simulink model "Four_DG_MG_PrimaryOnly"  (R2021b)
settings: Solver=ode23tb  StartTime=0.0  StopTime=5  RelTol=1e-3
model workspace (MAT data in the model file):
  Ts : Simulink.Parameter (value not decoded)
  secondary_on : Simulink.Parameter (value not decoded)
values from neighbouring files (symbols this model uses):
  a12 = 0    [Four_DG_MG_PrimaryOnlyScript.m]    (also in MPC_MG_script_raw_dmpc.m; MPC_MG_secondary_script.m)
  a14 = 0    [Four_DG_MG_PrimaryOnlyScript.m]    (also in MPC_MG_script_raw_dmpc.m; MPC_MG_secondary_script.m)
  a21 = 1    [Four_DG_MG_PrimaryOnlyScript.m]    (also in MPC_MG_script_raw_dmpc.m; MPC_MG_secondary_script.m)
  a23 = 0    [Four_DG_MG_PrimaryOnlyScript.m]    (also in MPC_MG_script_raw_dmpc.m; MPC_MG_secondary_script.m)
  a32 = 1    [Four_DG_MG_PrimaryOnlyScript.m]    (also in MPC_MG_script_raw_dmpc.m; MPC_MG_secondary_script.m)
  a34 = 0    [Four_DG_MG_PrimaryOnlyScript.m]    (also in MPC_MG_script_raw_dmpc.m; MPC_MG_secondary_script.m)
  a41 = 1    [Four_DG_MG_PrimaryOnlyScript.m]    (also in MPC_MG_script_raw_dmpc.m; MPC_MG_secondary_script.m)
  a43 = 0    [Four_DG_MG_PrimaryOnlyScript.m]    (also in MPC_MG_script_raw_dmpc.m; MPC_MG_secondary_script.m)
  b1v = 1    [Four_DG_MG_PrimaryOnlyScript.m]    (also in MPC_MG_script_raw_dmpc.m; MPC_MG_secondary_script.m; MPG_MG_July.m; MPG_MG_freq_script.m)
  b1w = 1    [Four_DG_MG_PrimaryOnlyScript.m]    (also in MPC_MG_script_raw_dmpc.m; MPC_MG_secondary_script.m; MPG_MG_July.m; MPG_MG_freq_script.m)
  b2v = 0    [Four_DG_MG_PrimaryOnlyScript.m]    (also in MPC_MG_script_raw_dmpc.m; MPC_MG_secondary_script.m; MPG_MG_July.m; MPG_MG_freq_script.m)
  b2w = 0    [Four_DG_MG_PrimaryOnlyScript.m]    (also in MPC_MG_script_raw_dmpc.m; MPC_MG_secondary_script.m; MPG_MG_July.m; MPG_MG_freq_script.m)
  b3v = 0    [Four_DG_MG_PrimaryOnlyScript.m]    (also in MPC_MG_script_raw_dmpc.m; MPC_MG_secondary_script.m; MPG_MG_July.m; MPG_MG_freq_script.m)
  b3w = 0    [Four_DG_MG_PrimaryOnlyScript.m]    (also in MPC_MG_script_raw_dmpc.m; MPC_MG_secondary_script.m; MPG_MG_July.m; MPG_MG_freq_script.m)
  b4v = 0    [Four_DG_MG_PrimaryOnlyScript.m]    (also in MPC_MG_script_raw_dmpc.m; MPC_MG_secondary_script.m; MPG_MG_July.m; MPG_MG_freq_script.m)
  b4w = 0    [Four_DG_MG_PrimaryOnlyScript.m]    (also in MPC_MG_script_raw_dmpc.m; MPC_MG_secondary_script.m; MPG_MG_July.m; MPG_MG_freq_script.m)
  C_f = 50e-6    (= 5e-05)    [Four_DG_MG_PrimaryOnlyScript.m]    (also in MPC_MG_script.m; MPC_MG_script_raw_dmpc.m; MPC_MG_secondary_script.m; MPG_MG_July.m)
  cf = 60    [Four_DG_MG_PrimaryOnlyScript.m]    (also in MPC_MG_script_raw_dmpc.m = 40; MPC_MG_secondary_script.m = 40; MPG_MG_July.m = 100; MPG_MG_freq_script.m = 100)
  cv = 60    [Four_DG_MG_PrimaryOnlyScript.m]    (also in MPC_MG_script_raw_dmpc.m = 40; MPC_MG_secondary_script.m = 40; MPG_MG_July.m = 100; MPG_MG_freq_script.m = 100)
  F = 1    [Four_DG_MG_PrimaryOnlyScript.m]    (also in dmpc.m = zeros(9,1))
  K_i1 = 420    [Four_DG_MG_PrimaryOnlyScript.m]
  K_i2 = K_i1    (= 420)    [Four_DG_MG_PrimaryOnlyScript.m]
  K_i3 = 390    [Four_DG_MG_PrimaryOnlyScript.m]
  K_i4 = K_i3    (= 390)    [Four_DG_MG_PrimaryOnlyScript.m]
  K_ii1 = 5e3    (= 5000)    [Four_DG_MG_PrimaryOnlyScript.m]
  K_ii2 = K_ii1    (= 5000)    [Four_DG_MG_PrimaryOnlyScript.m]
  K_ii3 = 16e3    (= 16000)    [Four_DG_MG_PrimaryOnlyScript.m]
  K_ii4 = K_ii3    (= 16000)    [Four_DG_MG_PrimaryOnlyScript.m]
  K_p1 = 0.1    [Four_DG_MG_PrimaryOnlyScript.m]
  K_p2 = K_p1    (= 0.1)    [Four_DG_MG_PrimaryOnlyScript.m]
  K_p3 = 0.05    [Four_DG_MG_PrimaryOnlyScript.m]
  K_p4 = K_p3    (= 0.05)    [Four_DG_MG_PrimaryOnlyScript.m]
  K_pi1 = 5    [Four_DG_MG_PrimaryOnlyScript.m]
  K_pi2 = K_pi1    (= 5)    [Four_DG_MG_PrimaryOnlyScript.m]
  K_pi3 = 10.5    [Four_DG_MG_PrimaryOnlyScript.m]
  K_pi4 = K_pi3    (= 10.5)    [Four_DG_MG_PrimaryOnlyScript.m]
  L_f = 1.35e-3    (= 0.00135)    [Four_DG_MG_PrimaryOnlyScript.m]    (also in MPC_MG_script.m; MPC_MG_script_raw_dmpc.m; MPC_MG_secondary_script.m; MPG_MG_July.m)
  L_in1 = 0.35e-3    (= 0.00035)    [Four_DG_MG_PrimaryOnlyScript.m]    (also in MPC_MG_script.m; MPC_MG_script_raw_dmpc.m; MPC_MG_secondary_script.m; MPG_MG_July.m)
  L_in2 = 0.35e-3    (= 0.00035)    [Four_DG_MG_PrimaryOnlyScript.m]    (also in MPC_MG_script.m; MPC_MG_script_raw_dmpc.m; MPC_MG_secondary_script.m; MPG_MG_July.m)
  L_in3 = 0.35e-3    (= 0.00035)    [Four_DG_MG_PrimaryOnlyScript.m]    (also in MPC_MG_script.m; MPC_MG_script_raw_dmpc.m; MPC_MG_secondary_script.m; MPG_MG_July.m)
  L_in4 = 0.35e-3    (= 0.00035)    [Four_DG_MG_PrimaryOnlyScript.m]    (also in MPC_MG_script.m; MPC_MG_script_raw_dmpc.m; MPC_MG_secondary_script.m; MPG_MG_July.m)
  lo_co = 0.2    [Four_DG_MG_PrimaryOnlyScript.m]    (also in MPC_MG_script.m = 0.05; MPC_MG_script_raw_dmpc.m; MPC_MG_secondary_script.m = 0.08; MPG_MG_July.m = 0.15)
  m_p1 = 9.4e-5/droopDivide    (= 9.4e-05)    [Four_DG_MG_PrimaryOnlyScript.m]    (also in MPC_MG_script.m; MPC_MG_script_raw_dmpc.m; MPC_MG_secondary_script.m; MPG_MG_July.m)
  m_p2 = 9.4e-5/droopDivide    (= 9.4e-05)    [Four_DG_MG_PrimaryOnlyScript.m]    (also in MPC_MG_script.m; MPC_MG_script_raw_dmpc.m; MPC_MG_secondary_script.m; MPG_MG_July.m)
  m_p3 = 12.5e-5/droopDivide    (= 0.000125)    [Four_DG_MG_PrimaryOnlyScript.m]    (also in MPC_MG_script.m; MPC_MG_script_raw_dmpc.m; MPC_MG_secondary_script.m; MPG_MG_July.m)
  m_p4 = 12.5e-5/droopDivide    (= 0.000125)    [Four_DG_MG_PrimaryOnlyScript.m]    (also in MPC_MG_script.m; MPC_MG_script_raw_dmpc.m; MPC_MG_secondary_script.m; MPG_MG_July.m)
  n_q1 = 1.3e-3/droopDivide2    (= 0.00013)    [Four_DG_MG_PrimaryOnlyScript.m]    (also in MPC_MG_script.m; MPC_MG_script_raw_dmpc.m; MPC_MG_secondary_script.m; MPG_MG_July.m)
  n_q2 = 1.3e-3/droopDivide2    (= 0.00013)    [Four_DG_MG_PrimaryOnlyScript.m]    (also in MPC_MG_script.m; MPC_MG_script_raw_dmpc.m; MPC_MG_secondary_script.m; MPG_MG_July.m)
  n_q3 = 1.5e-3/droopDivide2    (= 0.00015)    [Four_DG_MG_PrimaryOnlyScript.m]    (also in MPC_MG_script.m; MPC_MG_script_raw_dmpc.m; MPC_MG_secondary_script.m; MPG_MG_July.m)
  n_q4 = 1.5e-3/droopDivide2    (= 0.00015)    [Four_DG_MG_PrimaryOnlyScript.m]    (also in MPC_MG_script.m; MPC_MG_script_raw_dmpc.m; MPC_MG_secondary_script.m; MPG_MG_July.m)
  pq_gain = 3/2    (= 1.5)    [Four_DG_MG_PrimaryOnlyScript.m]
  R_f = 0.1    [Four_DG_MG_PrimaryOnlyScript.m]    (also in MPC_MG_script.m; MPC_MG_script_raw_dmpc.m; MPC_MG_secondary_script.m; MPG_MG_July.m)
  R_in1 = 0.03    [Four_DG_MG_PrimaryOnlyScript.m]    (also in MPC_MG_script.m; MPC_MG_script_raw_dmpc.m; MPC_MG_secondary_script.m; MPG_MG_July.m)
  R_in2 = 0.03    [Four_DG_MG_PrimaryOnlyScript.m]    (also in MPC_MG_script.m; MPC_MG_script_raw_dmpc.m; MPC_MG_secondary_script.m; MPG_MG_July.m)
  R_in3 = 0.03    [Four_DG_MG_PrimaryOnlyScript.m]    (also in MPC_MG_script.m; MPC_MG_script_raw_dmpc.m; MPC_MG_secondary_script.m; MPG_MG_July.m)
  R_in4 = 0.03    [Four_DG_MG_PrimaryOnlyScript.m]    (also in MPC_MG_script.m; MPC_MG_script_raw_dmpc.m; MPC_MG_secondary_script.m; MPG_MG_July.m)
  secondary = 1    [Four_DG_MG_PrimaryOnlyScript.m]
  secondary2 = 1    [Four_DG_MG_PrimaryOnlyScript.m]
  time_thresh = 0.6    [Four_DG_MG_PrimaryOnlyScript.m]    (also in MPC_MG_script_raw_dmpc.m = 1.5; MPC_MG_secondary_script.m = 2; MPG_MG_July.m = 0.5; MPG_MG_freq_script.m = 0.5)
  Ts = 10e-6    (= 1e-05)    [Four_DG_MG_PrimaryOnlyScript.m]    (also in MPC_MG_script.m; MPC_MG_script_raw_dmpc.m; MPC_MG_secondary_script.m; MPG_MG_July.m)
  V_nom = 220*sqrt(2)    [Four_DG_MG_PrimaryOnlyScript.m]    (also in MPC_MG_script.m; MPC_MG_script_raw_dmpc.m; MPC_MG_secondary_script.m; MPG_MG_July.m)
  Vdc = 600    [Four_DG_MG_PrimaryOnlyScript.m]    (also in MPC_MG_script.m; MPC_MG_script_raw_dmpc.m; MPC_MG_secondary_script.m; MPG_MG_July.m)
  w_nom = 2*pi*50    (= 314.159265359)    [Four_DG_MG_PrimaryOnlyScript.m]    (also in MPC_MG_script.m; MPC_MG_script_raw_dmpc.m; MPC_MG_secondary_script.m; MPG_MG_July.m)
undefined symbols (not defined in the file or in its folder): K_d
libraries: slpidlib x16, spsThreePhaseSeriesRLCBranchLib x15, spsabctodq0Lib x13, spsThreePhaseVIMeasurementLib x12, eeGeneralControl x8, spsOnDelayLib x8, spsPMUPLLBasedPositiveSequenceLib x4, eePwmGeneratorTwoLevel x4, spsdq0toabcLib x4, spsDCVoltageSourceLib x4, spsSeriesRLCBranchLib x4, spsTwoLevelConverterLib x4
(part 2 of 4)

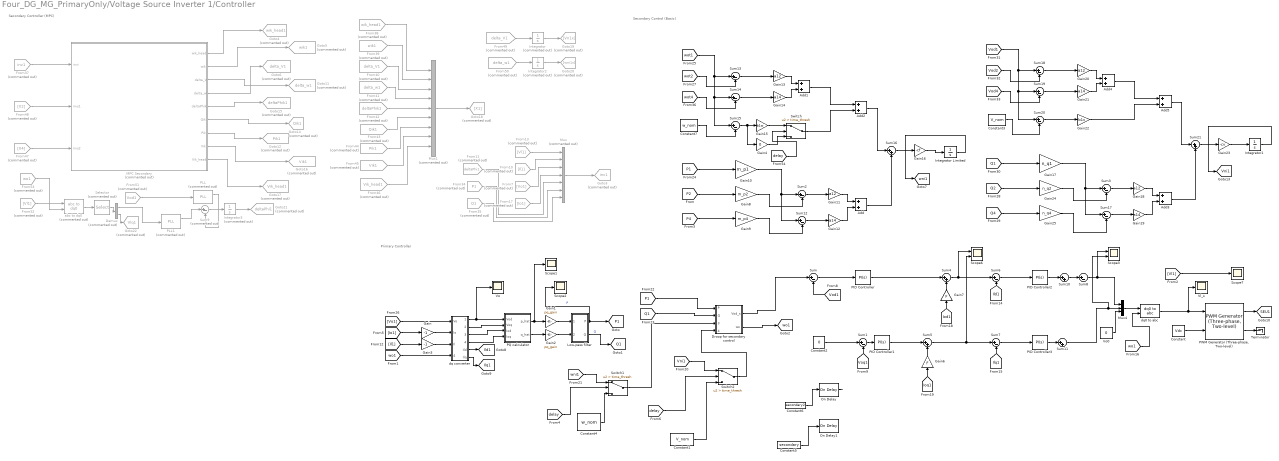
== system Four_DG_MG_PrimaryOnly/Voltage Source Inverter 1/Controller ==
  note: Secondary Controller (MPC)
  note: Secondary Control (Basic)
  note: Primary Controller
  Add{,1..5} (6 alike) : Sum
  Constant : Constant  Value=Vdc
  Constant1 : Constant  Value=V_nom
  Constant2 : Constant  Value=0
  Constant3 : Constant  Value=V_nom
  Constant4 : Constant  Value=w_nom
  Constant5 : Constant  Value=secondary
  Constant6 : Constant  Value=secondary2
  Constant7 : Constant  Value=w_nom
  Demux : Demux  Commented=on  Outputs=2
  Droop for secondary control : Subsystem
  From10 : From  Commented=on  GotoTag=Il1  TagVisibility=global
  From11 : From  Commented=on  GotoTag=deltaPhi1  TagVisibility=global
  From13 : From  Commented=on  GotoTag=Vl1  TagVisibility=global
  From17 : From  Commented=on  GotoTag=Io1  TagVisibility=global
  From34 : From  Commented=on  GotoTag=P1  TagVisibility=global
  From35 : From  Commented=on  GotoTag=Q1  TagVisibility=global
  From37 : From  Commented=on  GotoTag=inv1  TagVisibility=global
  From38 : From  Commented=on  GotoTag=wik_head1  TagVisibility=global
  From39 : From  Commented=on  GotoTag=wik1  TagVisibility=global
  From40 : From  Commented=on  GotoTag=delta_V1  TagVisibility=global
  From41 : From  Commented=on  GotoTag=delta_w1  TagVisibility=global
  From42 : From  Commented=on  GotoTag=deltaPhik1  TagVisibility=global
  From43 : From  Commented=on  GotoTag=Qik1  TagVisibility=global
  From44 : From  Commented=on  GotoTag=Pik1  TagVisibility=global
  From45 : From  Commented=on  GotoTag=Vik1  TagVisibility=global
  From46 : From  Commented=on  GotoTag=Vik_head1  TagVisibility=global
  From47 : From  Commented=on  GotoTag=X4
  From48 : From  Commented=on  GotoTag=X2
  From49 : From  Commented=on  GotoTag=delta_V1  TagVisibility=global
  From50 : From  Commented=on  GotoTag=delta_w1  TagVisibility=global
  From51 : From  Commented=on  GotoTag=Vod1  TagVisibility=global
  From52 : From  Commented=on  GotoTag=Vl1  TagVisibility=global
  From53 : From  Commented=on  GotoTag=wo1  TagVisibility=global
  From7 : From  Commented=on  GotoTag=Vo1  TagVisibility=global
  Gain : Gain  Gain=-1
  Gain1 : Gain  Gain=pq_gain
  Gain10 : Gain  Gain=m_p1
  Gain{11,13,18,20} (4 alike) : Gain  Gain=a12
  Gain{12,14,19,21} (4 alike) : Gain  Gain=a14
  Gain15 : Gain  Gain=b1w
  Gain16 : Gain  Gain=-cf
  Gain17 : Gain  Gain=n_q1
  Gain2 : Gain  Gain=pq_gain
  Gain22 : Gain  Gain=b1v
  Gain23 : Gain  Gain=-cv
  Gain24 : Gain  Gain=n_q2
  Gain25 : Gain  Gain=n_q4
  Gain3 : Gain  Gain=-1
  Gain4 : Gain  Gain=0
  Gain6 : Gain  Gain=F
  Gain7 : Gain  Gain=F
  Gain8 : Gain  Gain=m_p2
  Gain9 : Gain  Gain=m_p4
  Goto11 : Goto  Commented=on  GotoTag=delta_w1  TagVisibility=global
  Goto12 : Goto  Commented=on  GotoTag=Pik1  TagVisibility=global
  Goto14 : Goto  Commented=on  GotoTag=Qik1  TagVisibility=global
  Goto15 : Goto  Commented=on  GotoTag=deltaPhik1  TagVisibility=global
  Goto16 : Goto  Commented=on  GotoTag=Vik1  TagVisibility=global
  Goto17 : Goto  Commented=on  GotoTag=Vik_head1  TagVisibility=global
  Goto18 : Goto  Commented=on  GotoTag=X1
  Goto19 : Goto  Commented=on  GotoTag=Vn1x
  Goto20 : Goto  Commented=on  GotoTag=wni1x
  Goto21 : Goto  Commented=on  GotoTag=deltaPhi1  TagVisibility=global
  Goto22 : Goto  Commented=on  GotoTag=Vlq1  TagVisibility=global
  Goto3 : Goto  Commented=on  GotoTag=inv1  TagVisibility=global
  Goto4 : Goto  Commented=on  GotoTag=wik_head1  TagVisibility=global
  Goto5 : Goto  Commented=on  GotoTag=wik1  TagVisibility=global
  Goto6 : Goto  Commented=on  GotoTag=delta_V1  TagVisibility=global
  Integrator : Integrator  Commented=on
  Integrator Limited : Integrator  InitialCondition=50*2*pi  UpperSaturationLimit=51*2*pi  LowerSaturationLimit=50*2*pi
  Integrator1 : Integrator  InitialCondition=311  UpperSaturationLimit=373.35  LowerSaturationLimit=248.90
  Integrator2 : Integrator  Commented=on
  Integrator3 : Integrator  Commented=on
  Low-pass filter : Subsystem
  "MPC Secondary  " : MATLAB Function  Commented=on  TreatAsAtomicUnit=on
  Mux : Mux  Commented=on  Inputs=7
  Mux1 : Mux  Commented=on  Inputs=9
  Mux4 : Mux  Inputs=3
  On Delay : spsOnDelayLib/On Delay  DelayType=On delay  delay=4  ic=0  Ts=0
      settings: SourceProductBaseCode=PS
  On Delay1 : spsOnDelayLib/On Delay  DelayType=On delay  delay=4  ic=0  Ts=0
      settings: SourceProductBaseCode=PS
  PID Controller : slpidlib/PID Controller  Controller=PI  Form=Parallel  TimeDomain=Continuous-time  UseExternalTs=off  SampleTime=-1  IntegratorMethod=Forward Euler  FilterMethod=Forward Euler  ControllerParametersSource=internal  P=K_p1  I=K_i1  D=K_d  UseFilter=on  N=100  TunerSelectOption=Frequency Response Based  InitialConditionSource=internal  InitialConditionForIntegrator=0  InitialConditionForFilter=0  DifferentiatorICPrevScaledInput=0  ExternalReset=none  TrackingMode=off  Kt=1  LimitOutput=off  SatLimitsSource=internal  UpperSaturationLimit=50  LowerSaturationLimit=-50  LinearizeAsGain=on  AntiWindupMode=none  Kb=1  POutMin=[]  POutMax=[]  IOutMin=[]  IOutMax=[]  DOutMin=[]  DOutMax=[]  NOutMin=[]  NOutMax=[]  SumOutMin=[]  SumOutMax=[]  SaturationOutMin=[]  SaturationOutMax=[]  PParamMin=[]  PParamMax=[]  IParamMin=[]  IParamMax=[]  DParamMin=[]  DParamMax=[]  NParamMin=[]  NParamMax=[]  KbParamMin=[]  KbParamMax=[]  KtParamMin=[]  KtParamMax=[]  KbOutMin=[]  KbOutMax=[]  KtOutMin=[]  KtOutMax=[]  IntegratorOutMin=[]  IntegratorOutMax=[]  FilterOutMin=[]  FilterOutMax=[]  SumI1OutMin=[]  SumI1OutMax=[]  SumI2OutMin=[]  SumI2OutMax=[]  SumI3OutMin=[]  SumI3OutMax=[]  SumI4OutMin=[]  SumI4OutMax=[]  SumDOutMin=[]  SumDOutMax=[]  DifferentiatorOutMin=[]  DifferentiatorOutMax=[]  FilterDiffOutCoefMin=[]  FilterDiffOutCoefMax=[]  ReciprocalOutMin=[]  ReciprocalOutMax=[]  SumDenOutMin=[]  SumDenOutMax=[]  SumNumOutMin=[]  SumNumOutMax=[]  DivideOutMin=[]  DivideOutMax=[]  UdiffTsProdOutMin=[]  UdiffTsProdOutMax=[]  NTsProdOutMin=[]  NTsProdOutMax=[]  UintegralTsProdOutMin=[]  UintegralTsProdOutMax=[]  UngainTsProdOutMin=[]  UngainTsProdOutMax=[]  IntegratorContinuousStateAttributes=''  IntegratorStateMustResolveToSignalObject=off  IntegratorRTWStateStorageClass=Auto  FilterContinuousStateAttributes=''  FilterStateMustResolveToSignalObject=off  FilterRTWStateStorageClass=Auto  ParallelPVariant=InternalParameters  IdealPVariant=Disabled  IVariant=InternalParameters  DVariant=Disabled  IntegratorVariant=Continuous  SatVariant=Disabled  AWVariant=Passthrough  PCopyVariant=Disabled  TRVariant=Disabled  FdbkBlocksVariant=Forward  IdealPFdbkVariant=Disabled  SatFdbkVariant=Disabled  DerivativeFilterVariant=Disabled  NVariant=Disabled  NCopyVariant=Disabled_SignalSpec  FilterICVariant=Disabled  IntegratorICVariant=InternalICs  ExternalResetVariant=Disabled  TRSumVariant=Passthrough  SumFdbkVariant=Disabled  SumVariant=Sum_PI  TsampFilterVariant=InternalTs  TsampNgainVariant=Passthrough  TsampIntegralVariant=Passthrough  ExternalSaturationOutDataTypeStr=Inherit: Same as second input
  PID Controller1 : slpidlib/PID Controller  Controller=PI  Form=Parallel  TimeDomain=Continuous-time  UseExternalTs=off  SampleTime=-1  IntegratorMethod=Forward Euler  FilterMethod=Forward Euler  ControllerParametersSource=internal  P=K_p1  I=K_i1  D=K_d  UseFilter=on  N=100  TunerSelectOption=Frequency Response Based  InitialConditionSource=internal  InitialConditionForIntegrator=0  InitialConditionForFilter=0  DifferentiatorICPrevScaledInput=0  ExternalReset=none  TrackingMode=off  Kt=1  LimitOutput=off  SatLimitsSource=internal  UpperSaturationLimit=50  LowerSaturationLimit=-50  LinearizeAsGain=on  AntiWindupMode=none  Kb=1  POutMin=[]  POutMax=[]  IOutMin=[]  IOutMax=[]  DOutMin=[]  DOutMax=[]  NOutMin=[]  NOutMax=[]  SumOutMin=[]  SumOutMax=[]  SaturationOutMin=[]  SaturationOutMax=[]  PParamMin=[]  PParamMax=[]  IParamMin=[]  IParamMax=[]  DParamMin=[]  DParamMax=[]  NParamMin=[]  NParamMax=[]  KbParamMin=[]  KbParamMax=[]  KtParamMin=[]  KtParamMax=[]  KbOutMin=[]  KbOutMax=[]  KtOutMin=[]  KtOutMax=[]  IntegratorOutMin=[]  IntegratorOutMax=[]  FilterOutMin=[]  FilterOutMax=[]  SumI1OutMin=[]  SumI1OutMax=[]  SumI2OutMin=[]  SumI2OutMax=[]  SumI3OutMin=[]  SumI3OutMax=[]  SumI4OutMin=[]  SumI4OutMax=[]  SumDOutMin=[]  SumDOutMax=[]  DifferentiatorOutMin=[]  DifferentiatorOutMax=[]  FilterDiffOutCoefMin=[]  FilterDiffOutCoefMax=[]  ReciprocalOutMin=[]  ReciprocalOutMax=[]  SumDenOutMin=[]  SumDenOutMax=[]  SumNumOutMin=[]  SumNumOutMax=[]  DivideOutMin=[]  DivideOutMax=[]  UdiffTsProdOutMin=[]  UdiffTsProdOutMax=[]  NTsProdOutMin=[]  NTsProdOutMax=[]  UintegralTsProdOutMin=[]  UintegralTsProdOutMax=[]  UngainTsProdOutMin=[]  UngainTsProdOutMax=[]  IntegratorContinuousStateAttributes=''  IntegratorStateMustResolveToSignalObject=off  IntegratorRTWStateStorageClass=Auto  FilterContinuousStateAttributes=''  FilterStateMustResolveToSignalObject=off  FilterRTWStateStorageClass=Auto  ParallelPVariant=InternalParameters  IdealPVariant=Disabled  IVariant=InternalParameters  DVariant=Disabled  IntegratorVariant=Continuous  SatVariant=Disabled  AWVariant=Passthrough  PCopyVariant=Disabled  TRVariant=Disabled  FdbkBlocksVariant=Forward  IdealPFdbkVariant=Disabled  SatFdbkVariant=Disabled  DerivativeFilterVariant=Disabled  NVariant=Disabled  NCopyVariant=Disabled_SignalSpec  FilterICVariant=Disabled  IntegratorICVariant=InternalICs  ExternalResetVariant=Disabled  TRSumVariant=Passthrough  SumFdbkVariant=Disabled  SumVariant=Sum_PI  TsampFilterVariant=InternalTs  TsampNgainVariant=Passthrough  TsampIntegralVariant=Passthrough  ExternalSaturationOutDataTypeStr=Inherit: Same as second input
  PID Controller2 : slpidlib/PID Controller  Controller=PI  Form=Parallel  TimeDomain=Continuous-time  UseExternalTs=off  SampleTime=-1  IntegratorMethod=Forward Euler  FilterMethod=Forward Euler  ControllerParametersSource=internal  P=K_pi1  I=K_ii1  D=K_d  UseFilter=on  N=100  TunerSelectOption=Frequency Response Based  InitialConditionSource=internal  InitialConditionForIntegrator=0  InitialConditionForFilter=0  DifferentiatorICPrevScaledInput=0  ExternalReset=none  TrackingMode=off  Kt=1  LimitOutput=off  SatLimitsSource=internal  UpperSaturationLimit=inf  LowerSaturationLimit=-inf  LinearizeAsGain=on  AntiWindupMode=none  Kb=1  POutMin=[]  POutMax=[]  IOutMin=[]  IOutMax=[]  DOutMin=[]  DOutMax=[]  NOutMin=[]  NOutMax=[]  SumOutMin=[]  SumOutMax=[]  SaturationOutMin=[]  SaturationOutMax=[]  PParamMin=[]  PParamMax=[]  IParamMin=[]  IParamMax=[]  DParamMin=[]  DParamMax=[]  NParamMin=[]  NParamMax=[]  KbParamMin=[]  KbParamMax=[]  KtParamMin=[]  KtParamMax=[]  KbOutMin=[]  KbOutMax=[]  KtOutMin=[]  KtOutMax=[]  IntegratorOutMin=[]  IntegratorOutMax=[]  FilterOutMin=[]  FilterOutMax=[]  SumI1OutMin=[]  SumI1OutMax=[]  SumI2OutMin=[]  SumI2OutMax=[]  SumI3OutMin=[]  SumI3OutMax=[]  SumI4OutMin=[]  SumI4OutMax=[]  SumDOutMin=[]  SumDOutMax=[]  DifferentiatorOutMin=[]  DifferentiatorOutMax=[]  FilterDiffOutCoefMin=[]  FilterDiffOutCoefMax=[]  ReciprocalOutMin=[]  ReciprocalOutMax=[]  SumDenOutMin=[]  SumDenOutMax=[]  SumNumOutMin=[]  SumNumOutMax=[]  DivideOutMin=[]  DivideOutMax=[]  UdiffTsProdOutMin=[]  UdiffTsProdOutMax=[]  NTsProdOutMin=[]  NTsProdOutMax=[]  UintegralTsProdOutMin=[]  UintegralTsProdOutMax=[]  UngainTsProdOutMin=[]  UngainTsProdOutMax=[]  IntegratorContinuousStateAttributes=''  IntegratorStateMustResolveToSignalObject=off  IntegratorRTWStateStorageClass=Auto  FilterContinuousStateAttributes=''  FilterStateMustResolveToSignalObject=off  FilterRTWStateStorageClass=Auto  ParallelPVariant=InternalParameters  IdealPVariant=Disabled  IVariant=InternalParameters  DVariant=Disabled  IntegratorVariant=Continuous  SatVariant=Disabled  AWVariant=Passthrough  PCopyVariant=Disabled  TRVariant=Disabled  FdbkBlocksVariant=Forward  IdealPFdbkVariant=Disabled  SatFdbkVariant=Disabled  DerivativeFilterVariant=Disabled  NVariant=Disabled  NCopyVariant=Disabled_SignalSpec  FilterICVariant=Disabled  IntegratorICVariant=InternalICs  ExternalResetVariant=Disabled  TRSumVariant=Passthrough  SumFdbkVariant=Disabled  SumVariant=Sum_PI  TsampFilterVariant=InternalTs  TsampNgainVariant=Passthrough  TsampIntegralVariant=Passthrough  ExternalSaturationOutDataTypeStr=Inherit: Same as second input
  PID Controller3 : slpidlib/PID Controller  Controller=PI  Form=Parallel  TimeDomain=Continuous-time  UseExternalTs=off  SampleTime=-1  IntegratorMethod=Forward Euler  FilterMethod=Forward Euler  ControllerParametersSource=internal  P=K_pi1  I=K_ii1  D=K_d  UseFilter=on  N=100  TunerSelectOption=Frequency Response Based  InitialConditionSource=internal  InitialConditionForIntegrator=0  InitialConditionForFilter=0  DifferentiatorICPrevScaledInput=0  ExternalReset=none  TrackingMode=off  Kt=1  LimitOutput=off  SatLimitsSource=internal  UpperSaturationLimit=inf  LowerSaturationLimit=-inf  LinearizeAsGain=on  AntiWindupMode=none  Kb=1  POutMin=[]  POutMax=[]  IOutMin=[]  IOutMax=[]  DOutMin=[]  DOutMax=[]  NOutMin=[]  NOutMax=[]  SumOutMin=[]  SumOutMax=[]  SaturationOutMin=[]  SaturationOutMax=[]  PParamMin=[]  PParamMax=[]  IParamMin=[]  IParamMax=[]  DParamMin=[]  DParamMax=[]  NParamMin=[]  NParamMax=[]  KbParamMin=[]  KbParamMax=[]  KtParamMin=[]  KtParamMax=[]  KbOutMin=[]  KbOutMax=[]  KtOutMin=[]  KtOutMax=[]  IntegratorOutMin=[]  IntegratorOutMax=[]  FilterOutMin=[]  FilterOutMax=[]  SumI1OutMin=[]  SumI1OutMax=[]  SumI2OutMin=[]  SumI2OutMax=[]  SumI3OutMin=[]  SumI3OutMax=[]  SumI4OutMin=[]  SumI4OutMax=[]  SumDOutMin=[]  SumDOutMax=[]  DifferentiatorOutMin=[]  DifferentiatorOutMax=[]  FilterDiffOutCoefMin=[]  FilterDiffOutCoefMax=[]  ReciprocalOutMin=[]  ReciprocalOutMax=[]  SumDenOutMin=[]  SumDenOutMax=[]  SumNumOutMin=[]  SumNumOutMax=[]  DivideOutMin=[]  DivideOutMax=[]  UdiffTsProdOutMin=[]  UdiffTsProdOutMax=[]  NTsProdOutMin=[]  NTsProdOutMax=[]  UintegralTsProdOutMin=[]  UintegralTsProdOutMax=[]  UngainTsProdOutMin=[]  UngainTsProdOutMax=[]  IntegratorContinuousStateAttributes=''  IntegratorStateMustResolveToSignalObject=off  IntegratorRTWStateStorageClass=Auto  FilterContinuousStateAttributes=''  FilterStateMustResolveToSignalObject=off  FilterRTWStateStorageClass=Auto  ParallelPVariant=InternalParameters  IdealPVariant=Disabled  IVariant=InternalParameters  DVariant=Disabled  IntegratorVariant=Continuous  SatVariant=Disabled  AWVariant=Passthrough  PCopyVariant=Disabled  TRVariant=Disabled  FdbkBlocksVariant=Forward  IdealPFdbkVariant=Disabled  SatFdbkVariant=Disabled  DerivativeFilterVariant=Disabled  NVariant=Disabled  NCopyVariant=Disabled_SignalSpec  FilterICVariant=Disabled  IntegratorICVariant=InternalICs  ExternalResetVariant=Disabled  TRSumVariant=Passthrough  SumFdbkVariant=Disabled  SumVariant=Sum_PI  TsampFilterVariant=InternalTs  TsampNgainVariant=Passthrough  TsampIntegralVariant=Passthrough  ExternalSaturationOutDataTypeStr=Inherit: Same as second input
  PLL : spsPLLLib/PLL  Commented=on  Fmin=45  Par_Init=[0, 60]  ParK=[180, 3200, 1]  TcD=1e-4  MaxRateChangeFreq=12  FilterCutOffFreq=25  Ts=0  AGC=on
      settings: SourceProductBaseCode=PS
  PLL1 : spsPLLLib/PLL  Commented=on  Fmin=45  Par_Init=[0, 60]  ParK=[180, 3200, 1]  TcD=1e-4  MaxRateChangeFreq=12  FilterCutOffFreq=25  Ts=0  AGC=on
      settings: SourceProductBaseCode=PS
  PQ calculator : Subsystem
  "PWM Generator (Three-phase, Two-level)" : eePwmGeneratorTwoLevel/PWM Generator (Three-phase, Two-level)  PWMMode=Continuous PWM (CPWM)  CPWMMode=SPWM: sinusoidal PWM  DPWMMode=60 DPWM: 60 degree discontinuous PWM  fsw=f_c  Ts=Ts
      settings: SourceProductBaseCode=PS
  Scope1 : Scope
  Scope2 : Scope
  Scope3 : Scope  NumInputPorts=2
  Scope6 : Scope  NumInputPorts=2
  Scope7 : Scope
  Selector : Selector  Commented=on  InputPortWidth=3  IndexOptions=Index vector (dialog)  Indices=[1 2]  OutputSizes=1
  Sum{,1..3,6..8,12..15,17..20} (15 alike) : Sum  Inputs=|+-
  Sum{4..5,10..11,16,21} (6 alike) : Sum  Inputs=|++
  Sum9 : Sum  Commented=on  Inputs=|+-
  Switch : Switch  Criteria=u2 > Threshold  Threshold=time_thresh
  Switch1 : Switch  Criteria=u2 > Threshold  Threshold=time_thresh
  Switch2 : Switch  Criteria=u2 > Threshold  Threshold=time_thresh
  Terminator : Terminator
  Vl_s : Scope
  Vo : Scope
  Vo0 : Constant  Value=0
  abc to dq0 : spsabctodq0Lib/abc to dq0  Commented=on  Alignment=90 degrees behind phase A axis
  dq converter : Subsystem
  dq0 to abc : spsdq0toabcLib/dq0 to abc  Alignment=90 degrees behind phase A axis
  tag scope: Ild1=global, Ilq1=global, P1=global, Q1=global, SEU1=global, Vni1=global, wni1=global, wo1=global
  wires:
  dq converter/1(Vod) -> Vo/1, PQ calculator/1(Vod)
  [Vl1] -> Scope7/1
  [Io1] -> Gain/1
  Sum/1 -> PID Controller/1
  dq converter/6(Ilq) -> [Ilq1]
  Sum1/1 -> PID Controller1/1
  Sum7/1 -> PID Controller3/1
  [Voq1] -> Sum1/2
  dq converter/5(Ild) -> [Ild1]
  Mux4/1 -> dq0 to abc/1
  PID Controller1/1 -> Sum5/1
  Vo0/1 -> Mux4/3
  Sum6/1 -> PID Controller2/1
  PID Controller/1 -> Sum4/1
  PQ calculator/1(p_hat) -> Gain1/1, Scope1/1
  [Il1] -> Gain3/1
  [Vo1] -> dq converter/1(Vo)
  Sum11/1 -> Scope3/2, Mux4/2
  Gain6/1 -> Sum5/2
  dq converter/4(Ioq) -> PQ calculator/4(Ioq)
  "PWM Generator (Three-phase, Two-level)"/2 -> Terminator/1
  Sum5/1 -> Sum7/1, Scope6/2
  Constant/1 -> "PWM Generator (Three-phase, Two-level)"/2
  dq converter/3(Iod) -> PQ calculator/3(Iod)
  dq converter/2(Voq) -> PQ calculator/2(Voq)
  Sum8/1 -> Scope3/1, Mux4/1
  [Ioq1] -> Gain6/1
  dq0 to abc/1 -> Vl_s/1, "PWM Generator (Three-phase, Two-level)"/1
  [Ilq1] -> Sum7/2
  Gain1/1 -> Low-pass filter/1(p_hat)
  "PWM Generator (Three-phase, Two-level)"/1 -> [SEU1]
  [Ild1] -> Sum6/2
  [Vod1] -> Sum/2
  PQ calculator/2(q_hat) -> Gain2/1
  [wo1] -> dq0 to abc/2
  Low-pass filter/1(P) -> [P1], Scope2/1  "P"
  Droop for secondary control/2(wo) -> [wo1]
  [Q1] -> Droop for secondary control/2(Q)
  [P1] -> Droop for secondary control/1(P)
  Gain7/1 -> Sum4/2
  [Iod1] -> Gain7/1
  Sum4/1 -> Sum6/1, Scope6/1
  Gain2/1 -> Low-pass filter/2(q_hat)
  Low-pass filter/2(Q) -> [Q1]  "Q"
  Constant4/1 -> Switch1/3
  Constant1/1 -> Switch2/3
  [Vni1] -> Switch2/1
  [wni1] -> Switch1/1
  Switch2/1 -> Droop for secondary control/4(V_nom)
  [wo1] -> dq converter/4(wo1)
  Droop for secondary control/1(Vod_s) -> Sum/1
  PID Controller3/1 -> Sum11/1
  PID Controller2/1 -> Sum10/1
  Sum10/1 -> Sum8/1
  Constant2/1 -> Sum1/1
  Gain/1 -> dq converter/2(Io)
  Gain3/1 -> dq converter/3(Il)
  Add4/1 -> Add5/1
  Sum3/1 -> Gain18/1
  [Q1] -> Gain17/1
  Add2/1 -> Sum16/1
  Add5/1 -> Sum21/1
  [P1] -> Gain10/1
  Gain14/1 -> Add1/2
  Sum12/1 -> Gain12/1
  [Q4] -> Gain25/1
  Add3/1 -> Sum21/2
  Gain22/1 -> Add5/2
  Gain10/1 -> Sum12/1, Sum2/1
  Sum17/1 -> Gain19/1
  Gain13/1 -> Add1/1
  [Q2] -> Gain24/1
  [Vod1] -> Sum20/1, Sum19/1, Sum18/1
  [P4] -> Gain9/1
  Gain8/1 -> Sum2/2
  Sum16/1 -> Gain16/1
  Gain11/1 -> Add/1
  Sum18/1 -> Gain20/1
  Gain18/1 -> Add3/1
  [wot4] -> Sum14/2
  Sum14/1 -> Gain14/1
  Gain17/1 -> Sum17/1, Sum3/1
  Gain16/1 -> Integrator Limited/1
  [wot2] -> Sum13/2
  Gain25/1 -> Sum17/2
  Constant3/1 -> Sum20/2
  Integrator Limited/1 -> [wni1]
  Gain20/1 -> Add4/1
  [Vod2] -> Sum18/2
  Gain12/1 -> Add/2
  Gain23/1 -> Integrator1/1
  Sum13/1 -> Gain13/1
  Gain9/1 -> Sum12/2
  Sum19/1 -> Gain21/1
  Sum20/1 -> Gain22/1
  Integrator1/1 -> [Vni1]
  Gain24/1 -> Sum3/2
  Gain21/1 -> Add4/2
  Gain19/1 -> Add3/2
  Add/1 -> Sum16/2
  [P2] -> Gain8/1
  Add1/1 -> Add2/1
  Sum21/1 -> Gain23/1
  [Vod4] -> Sum19/2
  Sum2/1 -> Gain11/1
  Constant6/1 -> On Delay/1
  On Delay/1 -> ?
  Constant5/1 -> On Delay1/1
  [delay] -> Switch1/2
  [delay] -> Switch2/2
  [wot1] -> Sum15/1, Sum14/1, Sum13/1
  Switch1/1 -> Droop for secondary control/3(w_nom)
  From7/1 -> Mux/3
  From34/1 -> Mux/6
  From11/1 -> Mux/5
  From13/1 -> Mux/1
  Mux/1 -> Goto3/1
  From35/1 -> Mux/7
  From10/1 -> Mux/2
  From17/1 -> Mux/4
  From37/1 -> "MPC Secondary  "/1(invi)
  "MPC Secondary  "/1(wik_head) -> Goto4/1
  "MPC Secondary  "/2(wik) -> Goto5/1
  "MPC Secondary  "/4(delta_w) -> Goto6/1
  "MPC Secondary  "/3(delta_V) -> Goto11/1
  "MPC Secondary  "/5(deltaPhik) -> Goto15/1
  "MPC Secondary  "/6(Qik) -> Goto14/1
  "MPC Secondary  "/7(Pik) -> Goto12/1
  "MPC Secondary  "/8(Vik) -> Goto16/1
  "MPC Secondary  "/9(Vik_head) -> Goto17/1
  From42/1 -> Mux1/5
  From41/1 -> Mux1/4
  From40/1 -> Mux1/3
  From39/1 -> Mux1/2
  From38/1 -> Mux1/1
  From43/1 -> Mux1/6
  From44/1 -> Mux1/7
  From45/1 -> Mux1/8
  From46/1 -> Mux1/9
  Mux1/1 -> Goto18/1
  From48/1 -> "MPC Secondary  "/2(invj1)
  From47/1 -> "MPC Secondary  "/3(invj2)
  From49/1 -> Integrator/1
  From50/1 -> Integrator2/1
  Integrator/1 -> Goto19/1
  Integrator2/1 -> Goto20/1
  From51/1 -> PLL/1
  PLL/1 -> Sum9/2
  PLL1/1 -> Sum9/1
  Sum9/1 -> Integrator3/1
  Integrator3/1 -> Goto21/1
  From52/1 -> abc to dq0/1
  From53/1 -> abc to dq0/2
  abc to dq0/1 -> Selector/1
  Selector/1 -> Demux/1
  Demux/1 -> PLL1/1
  Demux/2 -> Goto22/1
  Constant7/1 -> Sum15/2
  Sum15/1 -> Gain4/1, Gain15/1
  Gain15/1 -> Switch/1
  Gain4/1 -> Switch/3
  [delay] -> Switch/2
  Switch/1 -> Add2/2

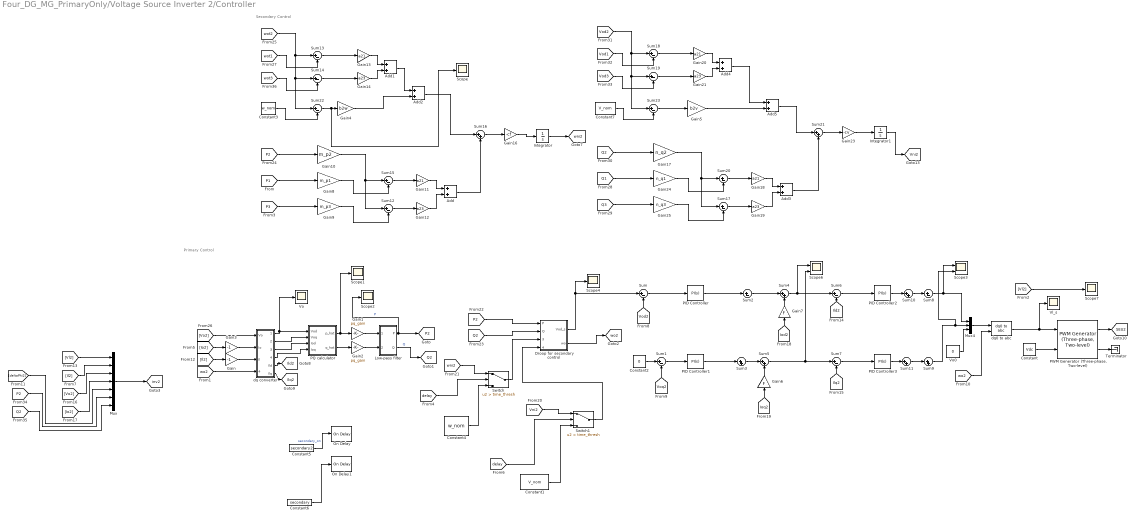
== system Four_DG_MG_PrimaryOnly/Voltage Source Inverter 2/Controller ==
  note: Secondary Control
  note: Primary Control
  Add{,1..5} (6 alike) : Sum
  Constant : Constant  Value=Vdc
  Constant1 : Constant  Value=V_nom
  Constant2 : Constant  Value=0
  Constant3 : Constant  Value=w_nom
  Constant4 : Constant  Value=w_nom
  Constant5 : Constant  Value=secondary2
  Constant6 : Constant  Value=secondary
  Constant7 : Constant  Value=V_nom
  Droop for secondary control : Subsystem
  Gain : Gain  Gain=-1
  Gain1 : Gain  Gain=pq_gain
  Gain10 : Gain  Gain=m_p2
  Gain{11,13,18,20} (4 alike) : Gain  Gain=a21
  Gain{12,14,19,21} (4 alike) : Gain  Gain=a23
  Gain16 : Gain  Gain=-cf
  Gain17 : Gain  Gain=n_q2
  Gain2 : Gain  Gain=pq_gain
  Gain23 : Gain  Gain=-cv
  Gain24 : Gain  Gain=n_q1
  Gain25 : Gain  Gain=n_q3
  Gain3 : Gain  Gain=-1
  Gain4 : Gain  Gain=b2w
  Gain5 : Gain  Gain=b2v
  Gain6 : Gain  Gain=F
  Gain7 : Gain  Gain=F
  Gain8 : Gain  Gain=m_p1
  Gain9 : Gain  Gain=m_p3
  Integrator : Integrator  InitialCondition=50*2*pi  UpperSaturationLimit=51*2*pi  LowerSaturationLimit=50*2*pi
  Integrator1 : Integrator  InitialCondition=311  UpperSaturationLimit=373.35  LowerSaturationLimit=248.90
  Low-pass filter : Subsystem
  Mux : Mux  Inputs=7
  Mux4 : Mux  Inputs=3
  On Delay : spsOnDelayLib/On Delay  DelayType=On delay  delay=4  ic=0  Ts=0
      settings: SourceProductBaseCode=PS
  On Delay1 : spsOnDelayLib/On Delay  DelayType=On delay  delay=4  ic=0  Ts=0
      settings: SourceProductBaseCode=PS
  PID Controller : slpidlib/PID Controller  Controller=PI  Form=Parallel  TimeDomain=Continuous-time  UseExternalTs=off  SampleTime=-1  IntegratorMethod=Forward Euler  FilterMethod=Forward Euler  ControllerParametersSource=internal  P=K_p2  I=K_i2  D=K_d  UseFilter=on  N=100  TunerSelectOption=Frequency Response Based  InitialConditionSource=internal  InitialConditionForIntegrator=0  InitialConditionForFilter=0  DifferentiatorICPrevScaledInput=0  ExternalReset=none  TrackingMode=off  Kt=1  LimitOutput=off  SatLimitsSource=internal  UpperSaturationLimit=50  LowerSaturationLimit=-50  LinearizeAsGain=on  AntiWindupMode=none  Kb=1  POutMin=[]  POutMax=[]  IOutMin=[]  IOutMax=[]  DOutMin=[]  DOutMax=[]  NOutMin=[]  NOutMax=[]  SumOutMin=[]  SumOutMax=[]  SaturationOutMin=[]  SaturationOutMax=[]  PParamMin=[]  PParamMax=[]  IParamMin=[]  IParamMax=[]  DParamMin=[]  DParamMax=[]  NParamMin=[]  NParamMax=[]  KbParamMin=[]  KbParamMax=[]  KtParamMin=[]  KtParamMax=[]  KbOutMin=[]  KbOutMax=[]  KtOutMin=[]  KtOutMax=[]  IntegratorOutMin=[]  IntegratorOutMax=[]  FilterOutMin=[]  FilterOutMax=[]  SumI1OutMin=[]  SumI1OutMax=[]  SumI2OutMin=[]  SumI2OutMax=[]  SumI3OutMin=[]  SumI3OutMax=[]  SumI4OutMin=[]  SumI4OutMax=[]  SumDOutMin=[]  SumDOutMax=[]  DifferentiatorOutMin=[]  DifferentiatorOutMax=[]  FilterDiffOutCoefMin=[]  FilterDiffOutCoefMax=[]  ReciprocalOutMin=[]  ReciprocalOutMax=[]  SumDenOutMin=[]  SumDenOutMax=[]  SumNumOutMin=[]  SumNumOutMax=[]  DivideOutMin=[]  DivideOutMax=[]  UdiffTsProdOutMin=[]  UdiffTsProdOutMax=[]  NTsProdOutMin=[]  NTsProdOutMax=[]  UintegralTsProdOutMin=[]  UintegralTsProdOutMax=[]  UngainTsProdOutMin=[]  UngainTsProdOutMax=[]  IntegratorContinuousStateAttributes=''  IntegratorStateMustResolveToSignalObject=off  IntegratorRTWStateStorageClass=Auto  FilterContinuousStateAttributes=''  FilterStateMustResolveToSignalObject=off  FilterRTWStateStorageClass=Auto  ParallelPVariant=InternalParameters  IdealPVariant=Disabled  IVariant=InternalParameters  DVariant=Disabled  IntegratorVariant=Continuous  SatVariant=Disabled  AWVariant=Passthrough  PCopyVariant=Disabled  TRVariant=Disabled  FdbkBlocksVariant=Forward  IdealPFdbkVariant=Disabled  SatFdbkVariant=Disabled  DerivativeFilterVariant=Disabled  NVariant=Disabled  NCopyVariant=Disabled_SignalSpec  FilterICVariant=Disabled  IntegratorICVariant=InternalICs  ExternalResetVariant=Disabled  TRSumVariant=Passthrough  SumFdbkVariant=Disabled  SumVariant=Sum_PI  TsampFilterVariant=InternalTs  TsampNgainVariant=Passthrough  TsampIntegralVariant=Passthrough  ExternalSaturationOutDataTypeStr=Inherit: Same as second input
  PID Controller1 : slpidlib/PID Controller  Controller=PI  Form=Parallel  TimeDomain=Continuous-time  UseExternalTs=off  SampleTime=-1  IntegratorMethod=Forward Euler  FilterMethod=Forward Euler  ControllerParametersSource=internal  P=K_p2  I=K_i2  D=K_d  UseFilter=on  N=100  TunerSelectOption=Frequency Response Based  InitialConditionSource=internal  InitialConditionForIntegrator=0  InitialConditionForFilter=0  DifferentiatorICPrevScaledInput=0  ExternalReset=none  TrackingMode=off  Kt=1  LimitOutput=off  SatLimitsSource=internal  UpperSaturationLimit=50  LowerSaturationLimit=-50  LinearizeAsGain=on  AntiWindupMode=none  Kb=1  POutMin=[]  POutMax=[]  IOutMin=[]  IOutMax=[]  DOutMin=[]  DOutMax=[]  NOutMin=[]  NOutMax=[]  SumOutMin=[]  SumOutMax=[]  SaturationOutMin=[]  SaturationOutMax=[]  PParamMin=[]  PParamMax=[]  IParamMin=[]  IParamMax=[]  DParamMin=[]  DParamMax=[]  NParamMin=[]  NParamMax=[]  KbParamMin=[]  KbParamMax=[]  KtParamMin=[]  KtParamMax=[]  KbOutMin=[]  KbOutMax=[]  KtOutMin=[]  KtOutMax=[]  IntegratorOutMin=[]  IntegratorOutMax=[]  FilterOutMin=[]  FilterOutMax=[]  SumI1OutMin=[]  SumI1OutMax=[]  SumI2OutMin=[]  SumI2OutMax=[]  SumI3OutMin=[]  SumI3OutMax=[]  SumI4OutMin=[]  SumI4OutMax=[]  SumDOutMin=[]  SumDOutMax=[]  DifferentiatorOutMin=[]  DifferentiatorOutMax=[]  FilterDiffOutCoefMin=[]  FilterDiffOutCoefMax=[]  ReciprocalOutMin=[]  ReciprocalOutMax=[]  SumDenOutMin=[]  SumDenOutMax=[]  SumNumOutMin=[]  SumNumOutMax=[]  DivideOutMin=[]  DivideOutMax=[]  UdiffTsProdOutMin=[]  UdiffTsProdOutMax=[]  NTsProdOutMin=[]  NTsProdOutMax=[]  UintegralTsProdOutMin=[]  UintegralTsProdOutMax=[]  UngainTsProdOutMin=[]  UngainTsProdOutMax=[]  IntegratorContinuousStateAttributes=''  IntegratorStateMustResolveToSignalObject=off  IntegratorRTWStateStorageClass=Auto  FilterContinuousStateAttributes=''  FilterStateMustResolveToSignalObject=off  FilterRTWStateStorageClass=Auto  ParallelPVariant=InternalParameters  IdealPVariant=Disabled  IVariant=InternalParameters  DVariant=Disabled  IntegratorVariant=Continuous  SatVariant=Disabled  AWVariant=Passthrough  PCopyVariant=Disabled  TRVariant=Disabled  FdbkBlocksVariant=Forward  IdealPFdbkVariant=Disabled  SatFdbkVariant=Disabled  DerivativeFilterVariant=Disabled  NVariant=Disabled  NCopyVariant=Disabled_SignalSpec  FilterICVariant=Disabled  IntegratorICVariant=InternalICs  ExternalResetVariant=Disabled  TRSumVariant=Passthrough  SumFdbkVariant=Disabled  SumVariant=Sum_PI  TsampFilterVariant=InternalTs  TsampNgainVariant=Passthrough  TsampIntegralVariant=Passthrough  ExternalSaturationOutDataTypeStr=Inherit: Same as second input
  PID Controller2 : slpidlib/PID Controller  Controller=PI  Form=Parallel  TimeDomain=Continuous-time  UseExternalTs=off  SampleTime=-1  IntegratorMethod=Forward Euler  FilterMethod=Forward Euler  ControllerParametersSource=internal  P=K_pi2  I=K_ii2  D=K_d  UseFilter=on  N=100  TunerSelectOption=Frequency Response Based  InitialConditionSource=internal  InitialConditionForIntegrator=0  InitialConditionForFilter=0  DifferentiatorICPrevScaledInput=0  ExternalReset=none  TrackingMode=off  Kt=1  LimitOutput=off  SatLimitsSource=internal  UpperSaturationLimit=inf  LowerSaturationLimit=-inf  LinearizeAsGain=on  AntiWindupMode=none  Kb=1  POutMin=[]  POutMax=[]  IOutMin=[]  IOutMax=[]  DOutMin=[]  DOutMax=[]  NOutMin=[]  NOutMax=[]  SumOutMin=[]  SumOutMax=[]  SaturationOutMin=[]  SaturationOutMax=[]  PParamMin=[]  PParamMax=[]  IParamMin=[]  IParamMax=[]  DParamMin=[]  DParamMax=[]  NParamMin=[]  NParamMax=[]  KbParamMin=[]  KbParamMax=[]  KtParamMin=[]  KtParamMax=[]  KbOutMin=[]  KbOutMax=[]  KtOutMin=[]  KtOutMax=[]  IntegratorOutMin=[]  IntegratorOutMax=[]  FilterOutMin=[]  FilterOutMax=[]  SumI1OutMin=[]  SumI1OutMax=[]  SumI2OutMin=[]  SumI2OutMax=[]  SumI3OutMin=[]  SumI3OutMax=[]  SumI4OutMin=[]  SumI4OutMax=[]  SumDOutMin=[]  SumDOutMax=[]  DifferentiatorOutMin=[]  DifferentiatorOutMax=[]  FilterDiffOutCoefMin=[]  FilterDiffOutCoefMax=[]  ReciprocalOutMin=[]  ReciprocalOutMax=[]  SumDenOutMin=[]  SumDenOutMax=[]  SumNumOutMin=[]  SumNumOutMax=[]  DivideOutMin=[]  DivideOutMax=[]  UdiffTsProdOutMin=[]  UdiffTsProdOutMax=[]  NTsProdOutMin=[]  NTsProdOutMax=[]  UintegralTsProdOutMin=[]  UintegralTsProdOutMax=[]  UngainTsProdOutMin=[]  UngainTsProdOutMax=[]  IntegratorContinuousStateAttributes=''  IntegratorStateMustResolveToSignalObject=off  IntegratorRTWStateStorageClass=Auto  FilterContinuousStateAttributes=''  FilterStateMustResolveToSignalObject=off  FilterRTWStateStorageClass=Auto  ParallelPVariant=InternalParameters  IdealPVariant=Disabled  IVariant=InternalParameters  DVariant=Disabled  IntegratorVariant=Continuous  SatVariant=Disabled  AWVariant=Passthrough  PCopyVariant=Disabled  TRVariant=Disabled  FdbkBlocksVariant=Forward  IdealPFdbkVariant=Disabled  SatFdbkVariant=Disabled  DerivativeFilterVariant=Disabled  NVariant=Disabled  NCopyVariant=Disabled_SignalSpec  FilterICVariant=Disabled  IntegratorICVariant=InternalICs  ExternalResetVariant=Disabled  TRSumVariant=Passthrough  SumFdbkVariant=Disabled  SumVariant=Sum_PI  TsampFilterVariant=InternalTs  TsampNgainVariant=Passthrough  TsampIntegralVariant=Passthrough  ExternalSaturationOutDataTypeStr=Inherit: Same as second input
  PID Controller3 : slpidlib/PID Controller  Controller=PI  Form=Parallel  TimeDomain=Continuous-time  UseExternalTs=off  SampleTime=-1  IntegratorMethod=Forward Euler  FilterMethod=Forward Euler  ControllerParametersSource=internal  P=K_pi2  I=K_ii2  D=K_d  UseFilter=on  N=100  TunerSelectOption=Frequency Response Based  InitialConditionSource=internal  InitialConditionForIntegrator=0  InitialConditionForFilter=0  DifferentiatorICPrevScaledInput=0  ExternalReset=none  TrackingMode=off  Kt=1  LimitOutput=off  SatLimitsSource=internal  UpperSaturationLimit=inf  LowerSaturationLimit=-inf  LinearizeAsGain=on  AntiWindupMode=none  Kb=1  POutMin=[]  POutMax=[]  IOutMin=[]  IOutMax=[]  DOutMin=[]  DOutMax=[]  NOutMin=[]  NOutMax=[]  SumOutMin=[]  SumOutMax=[]  SaturationOutMin=[]  SaturationOutMax=[]  PParamMin=[]  PParamMax=[]  IParamMin=[]  IParamMax=[]  DParamMin=[]  DParamMax=[]  NParamMin=[]  NParamMax=[]  KbParamMin=[]  KbParamMax=[]  KtParamMin=[]  KtParamMax=[]  KbOutMin=[]  KbOutMax=[]  KtOutMin=[]  KtOutMax=[]  IntegratorOutMin=[]  IntegratorOutMax=[]  FilterOutMin=[]  FilterOutMax=[]  SumI1OutMin=[]  SumI1OutMax=[]  SumI2OutMin=[]  SumI2OutMax=[]  SumI3OutMin=[]  SumI3OutMax=[]  SumI4OutMin=[]  SumI4OutMax=[]  SumDOutMin=[]  SumDOutMax=[]  DifferentiatorOutMin=[]  DifferentiatorOutMax=[]  FilterDiffOutCoefMin=[]  FilterDiffOutCoefMax=[]  ReciprocalOutMin=[]  ReciprocalOutMax=[]  SumDenOutMin=[]  SumDenOutMax=[]  SumNumOutMin=[]  SumNumOutMax=[]  DivideOutMin=[]  DivideOutMax=[]  UdiffTsProdOutMin=[]  UdiffTsProdOutMax=[]  NTsProdOutMin=[]  NTsProdOutMax=[]  UintegralTsProdOutMin=[]  UintegralTsProdOutMax=[]  UngainTsProdOutMin=[]  UngainTsProdOutMax=[]  IntegratorContinuousStateAttributes=''  IntegratorStateMustResolveToSignalObject=off  IntegratorRTWStateStorageClass=Auto  FilterContinuousStateAttributes=''  FilterStateMustResolveToSignalObject=off  FilterRTWStateStorageClass=Auto  ParallelPVariant=InternalParameters  IdealPVariant=Disabled  IVariant=InternalParameters  DVariant=Disabled  IntegratorVariant=Continuous  SatVariant=Disabled  AWVariant=Passthrough  PCopyVariant=Disabled  TRVariant=Disabled  FdbkBlocksVariant=Forward  IdealPFdbkVariant=Disabled  SatFdbkVariant=Disabled  DerivativeFilterVariant=Disabled  NVariant=Disabled  NCopyVariant=Disabled_SignalSpec  FilterICVariant=Disabled  IntegratorICVariant=InternalICs  ExternalResetVariant=Disabled  TRSumVariant=Passthrough  SumFdbkVariant=Disabled  SumVariant=Sum_PI  TsampFilterVariant=InternalTs  TsampNgainVariant=Passthrough  TsampIntegralVariant=Passthrough  ExternalSaturationOutDataTypeStr=Inherit: Same as second input
  PQ calculator : Subsystem
  "PWM Generator (Three-phase, Two-level)" : eePwmGeneratorTwoLevel/PWM Generator (Three-phase, Two-level)  PWMMode=Continuous PWM (CPWM)  CPWMMode=SPWM: sinusoidal PWM  DPWMMode=60 DPWM: 60 degree discontinuous PWM  fsw=f_c  Ts=Ts
      settings: SourceProductBaseCode=PS
  Scope{,1..2,4,7} (5 alike) : Scope
  Scope3 : Scope  NumInputPorts=2
  Scope6 : Scope  NumInputPorts=2
  Sum{,1..2,6..8,12..15,17..20,22..23} (16 alike) : Sum  Inputs=|+-
  Sum{3..5,9..11,16,21} (8 alike) : Sum  Inputs=|++
  Switch : Switch  Criteria=u2 > Threshold  Threshold=time_thresh
  Switch1 : Switch  Criteria=u2 > Threshold  Threshold=time_thresh
  Terminator : Terminator
  Vl_s : Scope
  Vo : Scope
  Vo0 : Constant  Value=0
  dq converter : Subsystem
  dq0 to abc : spsdq0toabcLib/dq0 to abc  Alignment=90 degrees behind phase A axis
  tag scope: Ild2=global, Ilq2=global, P2=global, Q2=global, SEU2=global, Vni2=global, inv2=global, wni2=global, wo2=global
  wires:
  dq converter/1(Vod) -> Vo/1, PQ calculator/1(Vod)
  ? -> Sum3/2
  [Vl2] -> Scope7/1
  ? -> Sum2/2
  [Io2] -> Gain3/1
  Sum/1 -> PID Controller/1
  dq converter/6(Ilq) -> [Ilq2]
  Sum1/1 -> PID Controller1/1
  Sum7/1 -> PID Controller3/1
  [Voq2] -> Sum1/2
  dq converter/5(Ild) -> [Ild2]
  Mux4/1 -> dq0 to abc/1
  PID Controller/1 -> Sum2/1
  PID Controller1/1 -> Sum3/1
  Vo0/1 -> Mux4/3
  Sum6/1 -> PID Controller2/1
  Sum2/1 -> Sum4/1
  PQ calculator/1(p_hat) -> Gain1/1, Scope1/1
  [Il2] -> Gain/1
  [Vo2] -> dq converter/1(Vo)
  Sum9/1 -> Scope3/2, Mux4/2
  Gain6/1 -> Sum5/2
  dq converter/4(Ioq) -> PQ calculator/4(Ioq)
  "PWM Generator (Three-phase, Two-level)"/2 -> Terminator/1
  Sum5/1 -> Scope6/2, Sum7/1
  Constant/1 -> "PWM Generator (Three-phase, Two-level)"/2
  dq converter/3(Iod) -> PQ calculator/3(Iod)
  dq converter/2(Voq) -> PQ calculator/2(Voq)
  Sum8/1 -> Scope3/1, Mux4/1
  [Ioq2] -> Gain6/1
  dq0 to abc/1 -> Vl_s/1, "PWM Generator (Three-phase, Two-level)"/1
  [Ilq2] -> Sum7/2
  Gain1/1 -> Low-pass filter/1(p_hat)
  "PWM Generator (Three-phase, Two-level)"/1 -> [SEU2]
  [Ild2] -> Sum6/2
  [Vod2] -> Sum/2
  PQ calculator/2(q_hat) -> Gain2/1
  [wo2] -> dq0 to abc/2
  Low-pass filter/1(P) -> [P2], Scope2/1  "P"
  [Q2] -> Droop for secondary control/2(Q)
  [P2] -> Droop for secondary control/1(P)
  Gain7/1 -> Sum4/2
  [Iod2] -> Gain7/1
  Sum4/1 -> Sum6/1, Scope6/1
  Sum3/1 -> Sum5/1
  Gain2/1 -> Low-pass filter/2(q_hat)
  Low-pass filter/2(Q) -> [Q2]  "Q"
  [wni2] -> Switch/1
  Constant4/1 -> Switch/3
  Switch/1 -> Droop for secondary control/3(w_nom)
  [Vni2] -> Switch1/1
  Constant1/1 -> Switch1/3
  Switch1/1 -> Droop for secondary control/4(V_nom)
  [wo2] -> dq converter/4(wo2)
  Droop for secondary control/1(Vod_s) -> Sum/1, Scope4/1
  Droop for secondary control/2(wo) -> [wo2]
  PID Controller3/1 -> Sum11/1
  Sum11/1 -> Sum9/1
  Sum10/1 -> Sum8/1
  PID Controller2/1 -> Sum10/1
  Constant2/1 -> Sum1/1
  Gain/1 -> dq converter/3(Il)
  Gain3/1 -> dq converter/2(Io)
  Gain21/1 -> Add4/2
  Sum21/1 -> Gain23/1
  [Q3] -> Gain25/1
  [Vod3] -> Sum19/2
  Gain19/1 -> Add3/2
  [wot2] -> Sum22/1, Sum14/1, Sum13/1
  [Q1] -> Gain24/1
  [wot1] -> Sum13/2
  Integrator/1 -> [wni2]
  Sum18/1 -> Gain20/1
  Sum20/1 -> Gain18/1
  Gain20/1 -> Add4/1
  Gain11/1 -> Add/1
  Gain25/1 -> Sum17/2
  Sum19/1 -> Gain21/1
  [Vod1] -> Sum18/2
  Gain24/1 -> Sum20/2
  Gain16/1 -> Integrator/1
  Sum15/1 -> Gain11/1
  [P3] -> Gain9/1
  Gain9/1 -> Sum12/2
  Gain23/1 -> Integrator1/1
  Sum17/1 -> Gain19/1
  Add/1 -> Sum16/2
  [wot3] -> Sum14/2
  Sum12/1 -> Gain12/1
  Integrator1/1 -> [Vni2]
  Gain8/1 -> Sum15/2
  Gain12/1 -> Add/2
  [Q2] -> Gain17/1
  [P2] -> Gain10/1
  Gain14/1 -> Add1/2
  Sum14/1 -> Gain14/1
  Sum16/1 -> Gain16/1
  [P1] -> Gain8/1
  Gain13/1 -> Add1/1
  Gain10/1 -> Sum12/1, Sum15/1
  [Vod2] -> Sum23/1, Sum19/1, Sum18/1
  Gain18/1 -> Add3/1
  Gain17/1 -> Sum17/1, Sum20/1
  Add3/1 -> Sum21/2
  Sum13/1 -> Gain13/1
  Constant5/1 -> On Delay/1  "secondary_on"
  Constant6/1 -> On Delay1/1
  [delay] -> Switch/2
  [delay] -> Switch1/2
  Constant3/1 -> Sum22/2
  Sum22/1 -> Scope/1, Gain4/1
  Add1/1 -> Add2/1
  Gain4/1 -> Add2/2
  Add2/1 -> Sum16/1
  Constant7/1 -> Sum23/2
  Sum23/1 -> Gain5/1
  Gain5/1 -> Add5/2
  Add4/1 -> Add5/1
  Add5/1 -> Sum21/1
  [Vo2] -> Mux/3
  [P2] -> Mux/6
  [deltaPhi2] -> Mux/5
  [Vl2] -> Mux/1
  Mux/1 -> [inv2]
  [Q2] -> Mux/7
  [Il2] -> Mux/2
  [Io2] -> Mux/4
